simulink model "modelloCatenaAperta"  (R2021a)
settings: Solver=VariableStepAuto  StartTime=0.0  StopTime=10.0  RelTol=1e-3
values from neighbouring files (symbols this model uses):
  b = 0.1    [PID.m]    (also in Studio in frequenza.m; controlloPID.m; modello_CA.m)
  g = 9.8    [PID.m]    (also in Studio in frequenza.m; controlloPID.m; modello2.m = 9.81; modello_CA.m)
  i = 0.006    [PID.m]    (also in Studio in frequenza.m; controlloPID.m; modello_CA.m)
  M = 0.5    [PID.m]    (also in Studio in frequenza.m; controlloPID.m; modello2.m = 0.04; modello_CA.m)
  m = 0.2    [PID.m]    (also in Studio in frequenza.m; controlloPID.m; modello2.m = 0.06; modello_CA.m)
settings Model: Creator=adolfocafaro  LastModifiedBy=olegg

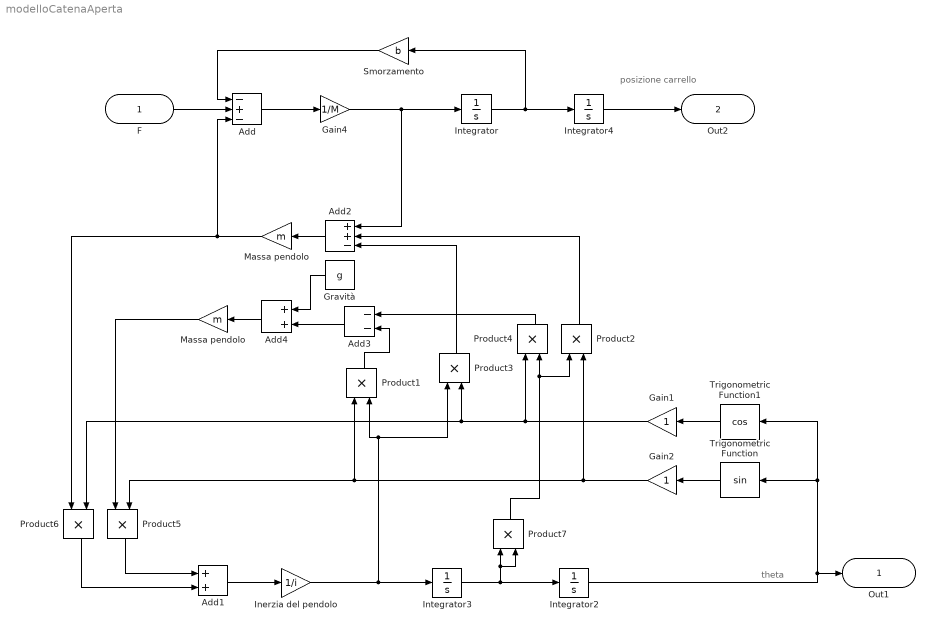
== system modelloCatenaAperta ==
  note: theta
  note: posizione carrello
  F : Inport
  Add : Sum  Inputs=-+-
  Add1 : Sum
  Add2 : Sum  Inputs=++-
  Add3 : Sum  Inputs=--
  Add4 : Sum
  Gain1 : Gain
  Gain2 : Gain
  Gain4 : Gain  Gain=1/M
  Gravità : Constant  Value=g
  Inerzia del pendolo : Gain  Gain=1/i
  Integrator{,2..4} (4 alike) : Integrator
  Massa pendolo : Gain  Gain=m
  "Massa pendolo " : Gain  Gain=m
  Product{1..7} (7 alike) : Product
  Smorzamento : Gain  Gain=b
  Trigonometric Function : Trigonometry
  Trigonometric Function1 : Trigonometry  Operator=cos
  Out1 : Outport
  Out2 : Outport  Port=2
  wires:
  F/1 -> Add/2
  Add/1 -> Gain4/1
  Gain4/1 -> Add2/1, Integrator/1
  Integrator/1 -> Smorzamento/1, Integrator4/1
  Smorzamento/1 -> Add/1
  Add2/1 -> Massa pendolo/1
  Add4/1 -> "Massa pendolo "/1
  Gravità/1 -> Add4/1
  Add3/1 -> Add4/2
  Product1/1 -> Add3/2
  Product4/1 -> Add3/1
  Product2/1 -> Add2/2
  Product3/1 -> Add2/3
  Product5/1 -> Add1/1
  Product6/1 -> Add1/2
  Add1/1 -> Inerzia del pendolo/1
  Massa pendolo/1 -> Add/3, Product6/1
  "Massa pendolo "/1 -> Product5/1
  Inerzia del pendolo/1 -> Integrator3/1, Product3/1, Product1/2
  Integrator3/1 -> Product7/2, Product7/1, Integrator2/1
  Integrator2/1 -> Out1/1, Trigonometric Function1/1, Trigonometric Function/1
  Trigonometric Function/1 -> Gain2/1
  Trigonometric Function1/1 -> Gain1/1
  Gain1/1 -> Product3/2, Product6/2, Product4/1
  Gain2/1 -> Product2/2, Product5/2, Product1/1
  Product7/1 -> Product2/1, Product4/2
  Integrator4/1 -> Out2/1
